simulink model "HapticSystem_Opspace"  (R2018a)
settings: Solver=VariableStepAuto  StartTime=0.0  StopTime=10.0  RelTol=1e-3
settings Model: Creator=augus  LastModifiedBy=augus

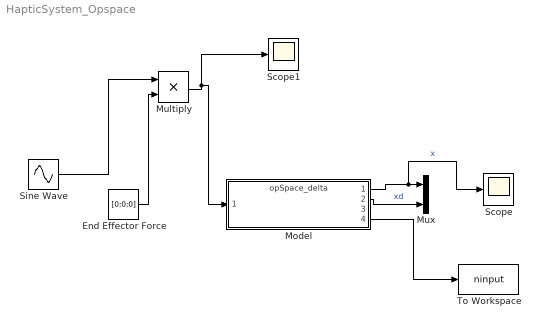
== system HapticSystem_Opspace ==
  End Effector Force : Constant  Value=[0;0;0]
  Model : ModelReference  ModelNameDialog=opSpace_delta  SimulationMode=Normal  Variant=on  ModelReferenceVersion=1.16
  Multiply : Product
  Mux : Mux  Inputs=2
  Scope : Scope
  Scope1 : Scope
  Sine Wave : Sin  Frequency=2*pi  SampleTime=0
  To Workspace : ToWorkspace  VariableName=ninput  SaveFormat=Timeseries  SampleTime=-1
  wires:
  Sine Wave/1 -> Multiply/1
  End Effector Force/1 -> Multiply/2
  Model/1 -> Scope/1, Mux/1  "x"
  Model/2 -> Mux/2  "xd"
  Multiply/1 -> Model/1, Scope1/1
  Model/4 -> To Workspace/1
